simulink model "uncertainty_disturbance_torques"  (Simulink 6.3)
settings: Solver=ode45  StartTime=0.0  StopTime=6179  RelTol=1e-3
libraries: components_lib x1
settings Model: Creator=mask02  LastModifiedBy=mnkr02  ExtModeAutoUpdateStatusClock=off  StrictBusMsg=None
settings DebuggingCC: CheckSSInitialOutputMsg=off

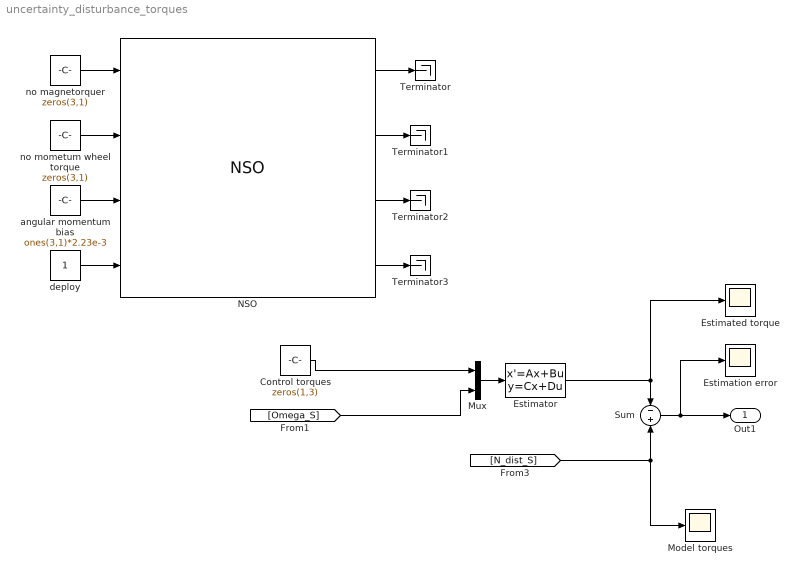
== system uncertainty_disturbance_torques ==
  Control torques : Constant  Value=zeros(1,3)
  Estimated torque : Scope
      settings: YMin=-2.5e-006  YMax=3e-006
  Estimation error : Scope
      settings: YMin=-2.5e-006  YMax=2.5e-006
  Estimator : StateSpace  A=[-1.8290 -0.0532 0.0523 23.6407 0 0; 0.0523 -1.8290 -0.0532 0 23.6407 0; -0.0790 0.0780 -2.2315 0 0 35.2113; -0.0706 -0.0021 0.0022 0 0 0; 0.0020 -0.0706 -0.0023 0 0 0; -0.0023 0.0022 -0.0706 0 0 0]  B=[-23.6407 0 0 1.8290 0.0005 0.0004; 0 -23.6407 0 0.0005 1.8290 0.0005; 0 0 -35.2113 0.0004 0.0005 2.2315; 0 0 0 0.0706 0.0021 -0.0022; 0 0 0 -0.0020 0.0706 0.0023; 0 0 0 0.0023 -0.0022 0.0706]  C=[zeros(3) eye(3)]  D=zeros(3,6)
  Model torques : Scope
      settings: YMin=-7.5e-007  YMax=7.5e-007  SaveName=ScopeData2
  Mux : Mux  Inputs=2
  NSO : components_lib/NSO  Tag=AAUSAT-II Model  Description=AAUSAT-II Model  r_com_s=[0.05 0.05 0.15]  sat_temp_start=0  r_com_s_deployed=[0.05 0.05 0.125]  mass_sc=3  Dim=[0.1 0.1 0.3]  inertia_c=[25 25 5]/1e3  inertia_d=Id  init_jd=2452315.56  q_s_c=[0 0 0 1]  q_init_s_i=q_att  w_init_s=[0.1 0.1 0.1]*0  Cd=cdrho  rho=1  enable_sensor_emulation=off  alb_emu_enabled=off  enable_dist=on
  Sum : Sum  Inputs=-|+
  Terminator{,1..3} (4 alike) : Terminator
  angular momentum bias : Constant  Value=ones(3,1)*2.23e-3
  deploy : Constant
  no magnetorquer : Constant  Value=zeros(3,1)
  no mometum wheel torque : Constant  Value=zeros(3,1)
  Out1 : Outport
  wires:
  deploy/1 -> NSO/4
  [Omega_S] -> Mux/2
  Control torques/1 -> Mux/1
  Estimator/1 -> Sum/1, Estimated torque/1
  [N_dist_S] -> Sum/2, Model torques/1
  Sum/1 -> Out1/1, Estimation error/1
  Mux/1 -> Estimator/1
  NSO/1 -> Terminator/1
  NSO/2 -> Terminator1/1
  NSO/3 -> Terminator2/1
  NSO/4 -> Terminator3/1
  no magnetorquer/1 -> NSO/1
  no mometum wheel torque/1 -> NSO/2
  angular momentum bias/1 -> NSO/3
